simulink model "model_sim"  (R2022a)
settings: Solver=VariableStepAuto  StartTime=0.0  StopTime=50  MaxStep=0.001  RelTol=1e-3
model workspace (MAT data in the model file):
  f_r = [100 100]
  j = 1
settings Model: Creator=tstef  LastModifiedBy=thomas
settings DebuggingCC: UnconnectedInputMsg=warning  UnconnectedOutputMsg=warning  UnconnectedLineMsg=warning
settings RTWCC: DLArmComputeVersion=19.05

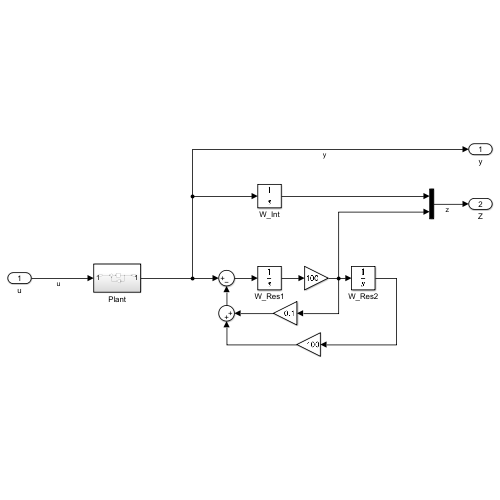
[thumbnail: Simulink's stored preview of the top-level diagram]
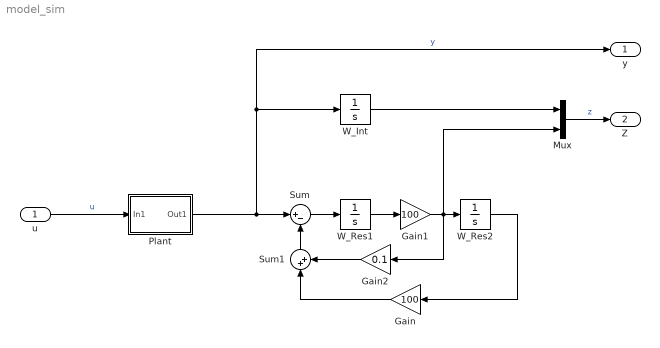
== system model_sim ==
  u : Inport
  Gain : Gain  Gain=100
  Gain1 : Gain  Gain=100
  Gain2 : Gain  Gain=0.1
  Mux : Mux  Inputs=2
  Plant : Subsystem
  Sum : Sum  Inputs=|+-
  Sum1 : Sum  Inputs=|++
  W_Int : Integrator
  W_Res1 : Integrator
  W_Res2 : Integrator
  y : Outport
  Z : Outport  Port=2
  wires:
  W_Res1/1 -> Gain1/1
  W_Res2/1 -> Gain/1
  Gain1/1 -> Mux/2, Gain2/1, W_Res2/1
  Sum/1 -> W_Res1/1
  Gain/1 -> Sum1/1
  Gain2/1 -> Sum1/2
  Sum1/1 -> Sum/2
  W_Int/1 -> Mux/1
  Mux/1 -> Z/1  "z"
  Plant/1(Out1) -> y/1, W_Int/1, Sum/1  "y"
  u/1 -> Plant/1(In1)  "u"

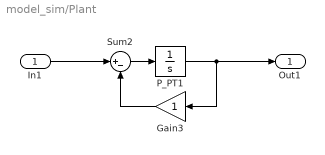
== system model_sim/Plant ==
  In1 : Inport
  Gain3 : Gain
  P_PT1 : Integrator
  Sum2 : Sum  Inputs=|+-
  Out1 : Outport
  wires:
  Sum2/1 -> P_PT1/1
  P_PT1/1 -> Out1/1, Gain3/1
  Gain3/1 -> Sum2/2
  In1/1 -> Sum2/1
